simulink model "modelJoystick"  (Simulink 7.0)
settings: Solver=ode23tb  StartTime=0.0  StopTime=1000.0  MaxStep=1  RelTol=1e-3
libraries: LemmingToolbox x7
settings Model: Creator=langmo  LastModifiedBy=langmo

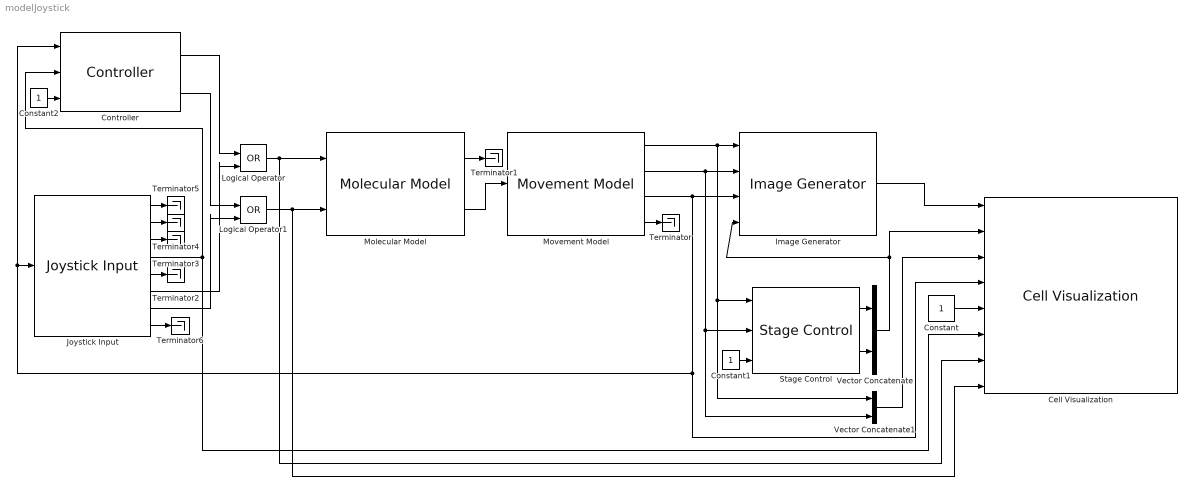
== system modelJoystick ==
  Cell Visualization : LemmingToolbox/Cell Visualization  SystemSampleTime=-1  outputFilename=fullModel.avi  imageDim=[1344,1024]  binning=2  maxNumCells=1  coneWidth=150  coneAngle=pi/4  pathLength=30  sampleTimes=[0.3, 0.1]
  Constant : Constant  OutDataTypeMode=uint32  OutDataType=sfix(16)  OutScaling=2^0
  Constant1 : Constant  OutDataType=sfix(16)  OutScaling=2^0
  Constant2 : Constant  OutDataTypeMode=boolean  OutDataType=sfix(16)  OutScaling=2^0
  Controller : LemmingToolbox/Controller  sampleTimes=[0.3, 0.1]  controller=@controllerHysteresis
  Image Generator : LemmingToolbox/Image Generator  binning=2  numCells=1  sampleTime=[0.3, 0.1]
  Joystick Input : LemmingToolbox/Joystick Input  SystemSampleTime=1  minMaxThresh=[0.05, 0.2]  sampleTimes=[0.1, 0]
  Logical Operator : Logic  Operator=OR  IconShape=distinctive  AllPortsSameDT=off  OutDataTypeMode=boolean
  Logical Operator1 : Logic  Operator=OR  IconShape=distinctive  AllPortsSameDT=off  OutDataTypeMode=boolean
  Molecular Model : LemmingToolbox/Molecular Model  molecModel=Spiro  controlledCheSpecies=CheY  cheSpeciesAttachedTo=CheX-PhyB & PIF3-Anker  asp=1e-3  useOrgParameters=on  CheX=20  AnkerProt=50  Anker=65
  Movement Model : LemmingToolbox/Movement Model  imageDim=[1344,1024]  binning=2  pixelSize=6.45 / 40  initialCondition=[0.5, 0.5, 0]  sampleTimes=[0.03, 0]
  Stage Control : LemmingToolbox/Stage Control  SystemSampleTime=-1  activate=on  controlMicroscope=off  cooldown=0  border=0.25  initialCondition=[0, 0]  sampleTimes=[0.3, 0.1]
  Terminator{,1..6} (7 alike) : Terminator
  Vector Concatenate : Concatenate  Mode=Vector  ConcatenateDimension=2
  Vector Concatenate1 : Concatenate  Mode=Multidimensional array  ConcatenateDimension=2
  wires:
  Stage Control/2 -> Vector Concatenate/2
  Stage Control/1 -> Vector Concatenate/1
  Controller/2 -> Logical Operator1/1
  Controller/1 -> Logical Operator/1
  Joystick Input/6 -> Logical Operator/2
  Logical Operator/1 -> Molecular Model/1, Cell Visualization/7
  Logical Operator1/1 -> Molecular Model/2, Cell Visualization/8
  Molecular Model/2 -> Movement Model/1
  Movement Model/1 -> Image Generator/1, Stage Control/1, Vector Concatenate1/1
  Movement Model/2 -> Image Generator/2, Stage Control/2, Vector Concatenate1/2
  Movement Model/3 -> Image Generator/3, Controller/1, Joystick Input/1, Cell Visualization/4
  Vector Concatenate/1 -> Image Generator/4, Cell Visualization/2
  Joystick Input/4 -> Controller/2, Cell Visualization/6
  Image Generator/1 -> Cell Visualization/1
  Vector Concatenate1/1 -> Cell Visualization/3
  Constant/1 -> Cell Visualization/5
  Movement Model/4 -> Terminator/1
  Molecular Model/1 -> Terminator1/1
  Joystick Input/5 -> Terminator2/1
  Joystick Input/3 -> Terminator3/1
  Joystick Input/2 -> Terminator4/1
  Joystick Input/1 -> Terminator5/1
  Joystick Input/7 -> Logical Operator1/2
  Constant1/1 -> Stage Control/3
  Constant2/1 -> Controller/3
  Joystick Input/8 -> Terminator6/1
